simulink model "Week3_Problem1"  (R2020a)
settings: Solver=FixedStepDiscrete  StartTime=0.0  StopTime=200  FixedStep=0.1  RelTol=1e-3
settings Model: Creator=tnradm  LastModifiedBy=tnradm

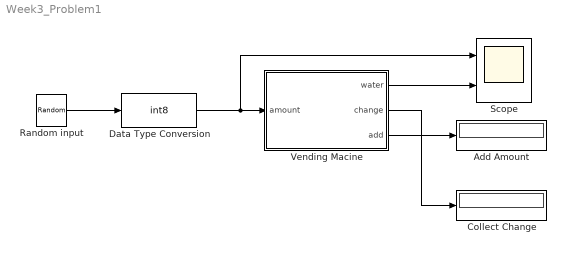
== system Week3_Problem1 ==
  Add Amount : Display
  Collect Change : Display
  Data Type Conversion : DataTypeConversion  OutDataTypeStr=int8  RndMeth=Nearest  SaturateOnIntegerOverflow=on
  Random input : UniformRandomNumber  Minimum=0  Maximum=100  Seed=337  SampleTime=10
  Scope : Scope  NumInputPorts=2
  Vending Macine : Stateflow chart  TreatAsAtomicUnit=on
  wires:
  Vending Macine/1(water) -> Scope/2
  Data Type Conversion/1 -> Scope/1, Vending Macine/1(amount)
  Vending Macine/2(change) -> Collect Change/1
  Vending Macine/3(add) -> Add Amount/1
  Random input/1 -> Data Type Conversion/1

== stateflow chart Week3_Problem1/Vending Macine ==
  state Start
  state Dispense_Change
  state Add_Amount
  state Dispense_Water
  (default) -> Start
  Add_Amount -> Start : {water=0}
  Start -> Dispense_Change [order 1] : [amount>10]{change=amount-10}
  Start -> Add_Amount [order 3] : [amount<10]{add=10-amount}
  Dispense_Water -> Start : {water=1}
  Start -> Dispense_Water [order 2] : [amount==10]{water=0}
  Dispense_Change -> Dispense_Water : {water=0}
  data: amount input; water output; change output; add output
